simulink model "failed_atempt"  (R2021a)
settings: Solver=VariableStepAuto  StartTime=0.0  StopTime=10.0  RelTol=1e-3
settings Model: Creator=Home  LastModifiedBy=Home

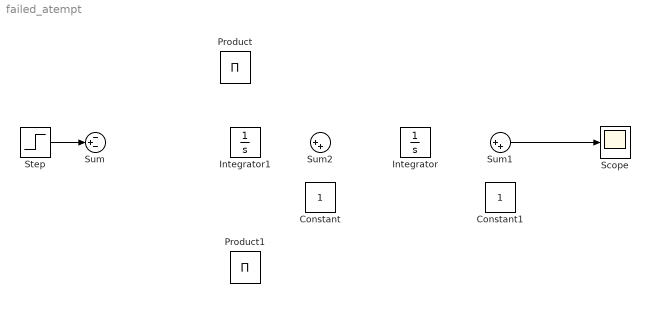
== system failed_atempt ==
  Constant : Constant
  Constant1 : Constant
  Integrator : Integrator
  Integrator1 : Integrator
  Product : Product  Inputs=1
  Product1 : Product  Inputs=1
  Scope : Scope
  Step : Step  After=50  SampleTime=0
  Sum : Sum  Inputs=-+-
  Sum1 : Sum  Inputs=|++
  Sum2 : Sum  Inputs=|++
  wires:
  Sum1/1 -> Scope/1
  Step/1 -> Sum/2
